simulink model "MSFartoystyring"  (Simulink 8.5)
settings: Solver=ode45  StartTime=tstart  StopTime=tstop  RelTol=1e-3
values from neighbouring files (symbols this model uses):
  c = normal_2(2) / normal_2(1)    [path_generation.m]    (also in run.m = 1; waypoints_collection.m = normal_2(obj.north) / normal_2(obj.east))
  not_use_beta_transform = 0    [run.m]
  not_use_speed_transform = 1    [run.m]
  psi0 = 0    [run.m]
  r0 = 0    [run.m]
  track = input(3)    [guidance_system.m]    (also in run.m = 1)
  tsamp = 10    [run.m]
  v0 = [6.63 0]'    [run.m]
undefined symbols (not defined in the file or in its folder): msfartoystyring
undefined symbols (not defined in the file): p0
settings Model: Creator=christh  LastModifiedBy=patrickf  ExtModeAutoUpdateStatusClock=off
settings OptimizationCC: InitFltsAndDblsToZero=on
settings DebuggingCC: SolverPrmCheckMsg=warning  FcnCallInpInsideContextMsg=UseLocalSettings

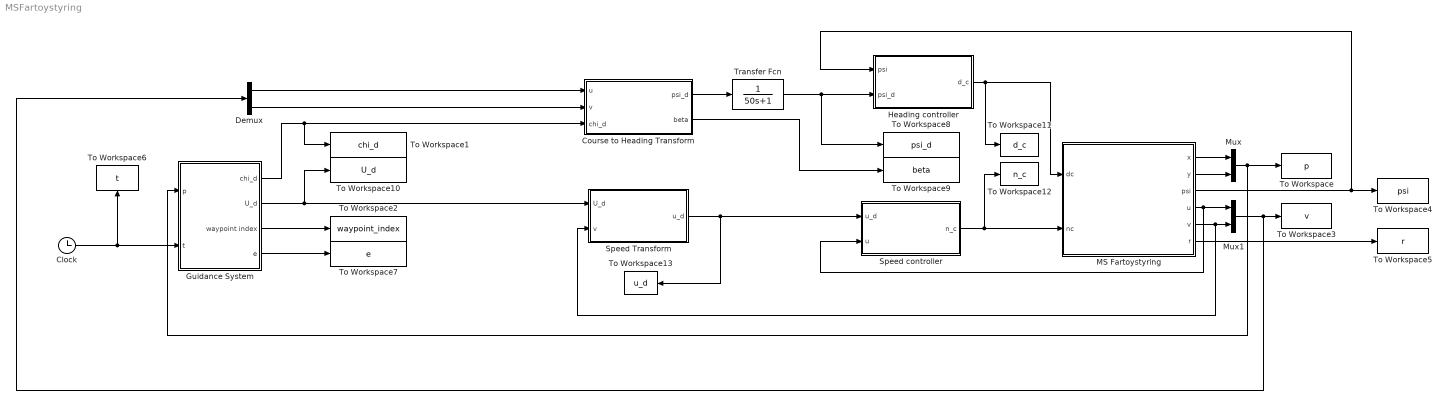
== system MSFartoystyring ==
  Clock : Clock
  Course to Heading Transform : Subsystem
  Demux : Demux  Outputs=2
  "Guidance System " : Subsystem
  Heading controller : Subsystem
  MS Fartoystyring : Subsystem  mask(MS Fartoystyring for Assignment 3 G&C){x0=p0(1), y0=p0(2), u0=v0(1), v0=v0(2), psi0=psi0, r0=r0, c=c}
      mask prompts: x0 "x(t0) (m)"; y0 "y(t0) (m)"; u0 "u(t0) (m/s)"; v0 "v(t0) (m/s)"; psi0 "psi(t0) (rad)"; r0 "r(t0) (rad/s)"; c "current (0 or 1)"
      mask help:
      | Block corresponding to Figure 1 in the assignment text. Gives the response of the ship.
      |
      | The design speed of MS Fartoystyring is u=8.23 m/s.
      |
      | Input:
      | dc: commanded rudder (rad), dmax=25*pi/180
      | nc: commanded shaft speed (rad/s), nmax=85*2*pi/60
      |
      | Output:
      | x: north pos (m)
      | y: east pos (m)
      | u: surge (m/s)
      | v: sway (m/s)
      | psi: heading (rad)
      | r: yaw (rad/s)
      mask Help: Comments, bugs and help requests can be directed to the TA. Email on course website.
  Mux : Mux  Inputs=2
  Mux1 : Mux  Inputs=2
  Speed Transform : Subsystem
  Speed controller : Subsystem
  To Workspace : ToWorkspace  VariableName=p  SampleTime=tsamp
  To Workspace1 : ToWorkspace  VariableName=chi_d  SampleTime=tsamp
  To Workspace10 : ToWorkspace  VariableName=U_d  SampleTime=tsamp
  To Workspace11 : ToWorkspace  VariableName=d_c  SampleTime=tsamp
  To Workspace12 : ToWorkspace  VariableName=n_c  SampleTime=tsamp
  To Workspace13 : ToWorkspace  VariableName=u_d  SampleTime=tsamp
  To Workspace2 : ToWorkspace  VariableName=waypoint_index  SampleTime=tsamp
  To Workspace3 : ToWorkspace  VariableName=v  SampleTime=tsamp
  To Workspace4 : ToWorkspace  VariableName=psi  SampleTime=tsamp
  To Workspace5 : ToWorkspace  VariableName=r  SampleTime=tsamp
  To Workspace6 : ToWorkspace  VariableName=t  SampleTime=tsamp
  To Workspace7 : ToWorkspace  VariableName=e  SampleTime=tsamp
  To Workspace8 : ToWorkspace  VariableName=psi_d  SampleTime=tsamp
  To Workspace9 : ToWorkspace  VariableName=beta  SampleTime=tsamp
  Transfer Fcn : TransferFcn  Denominator=[50 1]
  wires:
  Clock/1 -> To Workspace6/1, "Guidance System "/2(t)
  MS Fartoystyring/1(x) -> Mux/1
  MS Fartoystyring/2(y) -> Mux/2
  MS Fartoystyring/4(u) -> Speed controller/2(u), Mux1/1
  MS Fartoystyring/5(v) -> Speed Transform/2(v), Mux1/2
  Mux/1 -> To Workspace/1, "Guidance System "/1(p)
  Mux1/1 -> Demux/1, To Workspace3/1
  MS Fartoystyring/3(psi) -> Heading controller/1(psi), To Workspace4/1
  MS Fartoystyring/6(r) -> To Workspace5/1
  Heading controller/1(d_c) -> To Workspace11/1, MS Fartoystyring/1(dc)
  "Guidance System "/3(waypoint index) -> To Workspace2/1
  "Guidance System "/4(e) -> To Workspace7/1
  Course to Heading Transform/1(psi_d) -> Transfer Fcn/1
  Demux/1 -> Course to Heading Transform/1(u)
  Demux/2 -> Course to Heading Transform/2(v)
  Course to Heading Transform/2(beta) -> To Workspace9/1
  "Guidance System "/2(U_d) -> To Workspace10/1, Speed Transform/1(U_d)
  Speed Transform/1(u_d) -> To Workspace13/1, Speed controller/1(u_d)
  Speed controller/1(n_c) -> To Workspace12/1, MS Fartoystyring/2(nc)
  "Guidance System "/1(chi_d) -> To Workspace1/1, Course to Heading Transform/3(chi_d)
  Transfer Fcn/1 -> To Workspace8/1, Heading controller/2(psi_d)

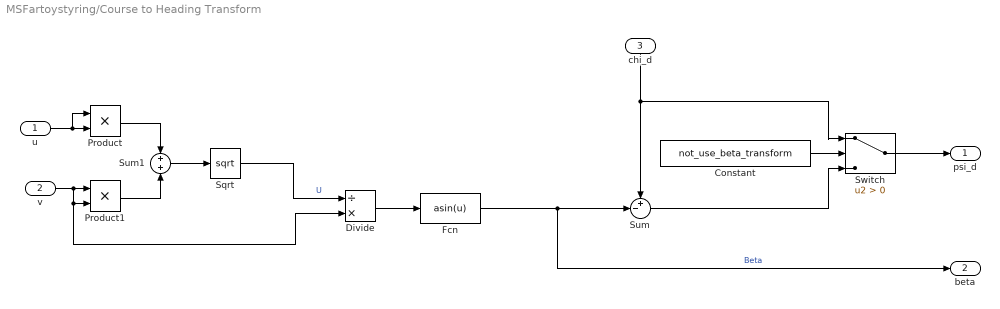
== system MSFartoystyring/Course to Heading Transform ==
  u : Inport
  v : Inport  Port=2
  chi_d : Inport  Port=3
  Constant : Constant  Value=not_use_beta_transform
  Divide : Product  Inputs=/*
  Fcn : Fcn  Expr=asin(u)
  Product : Product
  Product1 : Product
  Sqrt : Sqrt  SaturateOnIntegerOverflow=on
  Sum : Sum  Inputs=+-|
  Sum1 : Sum  Inputs=+|+
  Switch : Switch  Criteria=u2 > Threshold
  psi_d : Outport
  beta : Outport  Port=2
  wires:
  Fcn/1 -> beta/1, Sum/2  "Beta"
  Divide/1 -> Fcn/1
  chi_d/1 -> Sum/1, Switch/1
  v/1 -> Divide/2, Product1/2, Product1/1
  u/1 -> Product/1, Product/2
  Product/1 -> Sum1/1
  Product1/1 -> Sum1/2
  Sum1/1 -> Sqrt/1
  Sqrt/1 -> Divide/1  "U"
  Constant/1 -> Switch/2
  Switch/1 -> psi_d/1
  Sum/1 -> Switch/3

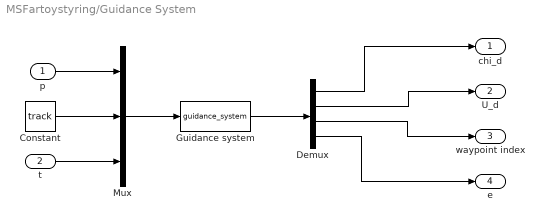
== system MSFartoystyring/Guidance System  ==
  p : Inport
  t : Inport  Port=2
  Constant : Constant  Value=track
  Demux : Demux
  Guidance system : MATLABFcn  MATLABFcn=guidance_system  Output1D=off
  Mux : Mux  Inputs=3
  chi_d : Outport
  U_d : Outport  Port=2
  waypoint index : Outport  Port=3
  e : Outport  Port=4
  wires:
  Guidance system/1 -> Demux/1
  Demux/2 -> U_d/1
  Demux/1 -> chi_d/1
  Demux/3 -> waypoint index/1
  Demux/4 -> e/1
  p/1 -> Mux/1
  Constant/1 -> Mux/2
  Mux/1 -> Guidance system/1
  t/1 -> Mux/3

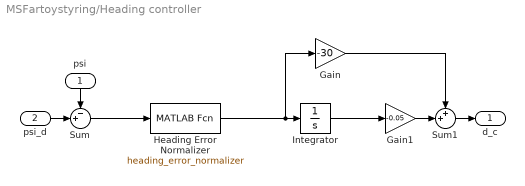
== system MSFartoystyring/Heading controller ==
  psi : Inport
  psi_d : Inport  Port=2
  Gain : Gain  Gain=-30
  Gain1 : Gain  Gain=-0.05
  Heading Error Normalizer : MATLABFcn  MATLABFcn=heading_error_normalizer
  Integrator : Integrator
  Sum : Sum  Inputs=-+|
  Sum1 : Sum  Inputs=++|
  d_c : Outport
  wires:
  Sum/1 -> Heading Error Normalizer/1
  psi/1 -> Sum/1
  Sum1/1 -> d_c/1
  psi_d/1 -> Sum/2
  Gain/1 -> Sum1/1
  Integrator/1 -> Gain1/1
  Gain1/1 -> Sum1/2
  Heading Error Normalizer/1 -> Integrator/1, Gain/1

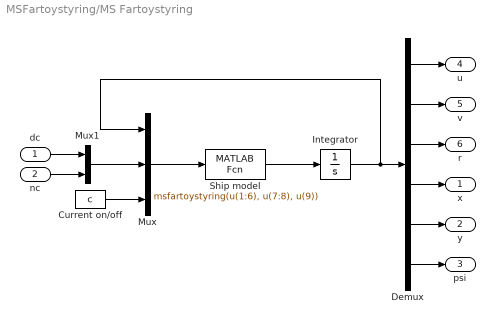
== system MSFartoystyring/MS Fartoystyring ==
  dc : Inport
  nc : Inport  Port=2
  Current on/off : Constant  Value=c
  Demux : Demux  Outputs=6
  Integrator : Integrator  InitialCondition=[u0 v0 r0 x0 y0 psi0]'
  Mux : Mux  Inputs=3
  Mux1 : Mux  Inputs=2
  Ship model : MATLABFcn  MATLABFcn=msfartoystyring(u(1:6), u(7:8), u(9))  OutputDimensions=6
  x : Outport
  y : Outport  Port=2
  psi : Outport  Port=3
  u : Outport  Port=4
  v : Outport  Port=5
  r : Outport  Port=6
  wires:
  Integrator/1 -> Mux/1, Demux/1
  Mux1/1 -> Mux/2
  dc/1 -> Mux1/1
  nc/1 -> Mux1/2
  Demux/1 -> u/1
  Demux/2 -> v/1
  Demux/3 -> r/1
  Demux/4 -> x/1
  Demux/5 -> y/1
  Demux/6 -> psi/1
  Current on/off/1 -> Mux/3
  Ship model/1 -> Integrator/1
  Mux/1 -> Ship model/1

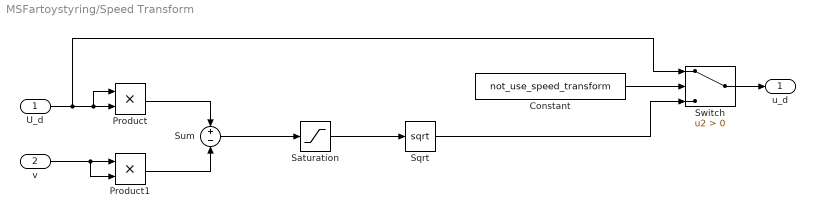
== system MSFartoystyring/Speed Transform ==
  U_d : Inport
  v : Inport  Port=2
  Constant : Constant  Value=not_use_speed_transform
  Product : Product
  Product1 : Product
  Saturation : Saturate  UpperLimit=Inf  LowerLimit=0
  Sqrt : Sqrt  SaturateOnIntegerOverflow=on
  Sum : Sum  Inputs=+|-
  Switch : Switch  Criteria=u2 > Threshold
  u_d : Outport
  wires:
  Product1/1 -> Sum/2
  v/1 -> Product1/2, Product1/1
  Sum/1 -> Saturation/1
  Product/1 -> Sum/1
  Saturation/1 -> Sqrt/1
  Constant/1 -> Switch/2
  Sqrt/1 -> Switch/3
  Switch/1 -> u_d/1
  U_d/1 -> Switch/1, Product/1, Product/2

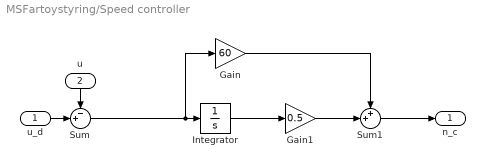
== system MSFartoystyring/Speed controller ==
  u_d : Inport
  u : Inport  Port=2
  Gain : Gain  Gain=60
  Gain1 : Gain  Gain=0.5
  Integrator : Integrator
  Sum : Sum  Inputs=-+|
  Sum1 : Sum  Inputs=++|
  n_c : Outport
  wires:
  u/1 -> Sum/1
  Sum1/1 -> n_c/1
  u_d/1 -> Sum/2
  Gain/1 -> Sum1/1
  Integrator/1 -> Gain1/1
  Gain1/1 -> Sum1/2
  Sum/1 -> Integrator/1, Gain/1
